simulink model "sim_Ex3"  (R2022b)
settings: Solver=FixedStepAuto  StartTime=0.0  StopTime=10.0  FixedStep=1e-3  RelTol=1e-3
values from neighbouring files (symbols this model uses):
  MassValue = mass(i)    [sim_Ex3_script.m]
settings Model: Creator=MAAM  LastModifiedBy=MAAM

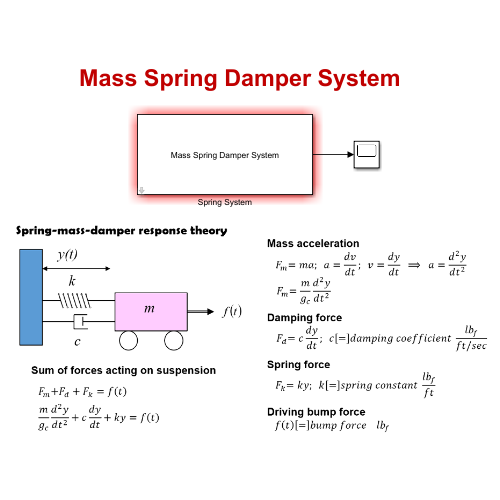
[thumbnail: Simulink's stored preview of the top-level diagram]
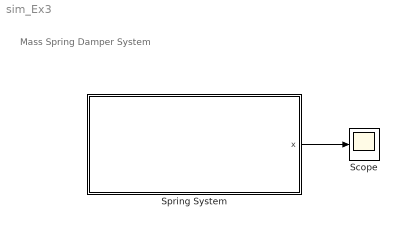
== system sim_Ex3 ==
  note: Mass Spring Damper System
  Scope : Scope
  Spring System : Subsystem  mask{m=MassValue, c=10, k=400, x0=1}
      mask prompts: m "Mass m"; c "Damping Coefficient c"; k "Spring constant k"; x0 "Init Distance x0"
      mask Display: fprintf('Mass Spring Damper System');
  wires:
  Spring System/1(x) -> Scope/1

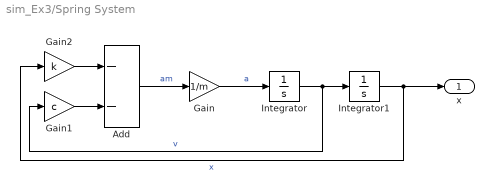
== system sim_Ex3/Spring System ==
  Add : Sum  Inputs=--
  Gain : Gain  Gain=1/m
  Gain1 : Gain  Gain=c
  Gain2 : Gain  Gain=k
  Integrator : Integrator
  Integrator1 : Integrator  InitialCondition=x0
  x : Outport
  wires:
  Gain2/1 -> Add/1
  Gain1/1 -> Add/2
  Gain/1 -> Integrator/1  "a"
  Add/1 -> Gain/1  "am"
  Integrator/1 -> Gain1/1, Integrator1/1  "v"
  Integrator1/1 -> Gain2/1, x/1  "x"
